simulink model "s_heli3d_Kalman_Filter"  (Simulink 7.7)
settings: Solver=ode1  StartTime=0.0  StopTime=70  FixedStep=0.007  RelTol=1e-3
values from neighbouring files (symbols this model uses):
  A = double(subs(J_a,{'x1','x2','x3','x4','x5','x6','u1','u2'},{x0(1),x0(2),x0(3),x0(4),x0(5),x0(6),u0(1),u0(2)}))    [linnlsys.m]    (also in o_lqi.m = A_lin)
  A_kal = Kest.a    [setup_lab_heli_3d_various_controler_with_Kalman_Filter.m]
  B = double(subs(J_b,{'x1','x2','x3','x4','x5','x6','u1','u2'},{x0(1),x0(2),x0(3),x0(4),x0(5),x0(6),u0(1),u0(2)}))    [linnlsys.m]    (also in o_lqi.m = B_lin)
  B_kal = Kest.b    [setup_lab_heli_3d_various_controler_with_Kalman_Filter.m]
  C_kal = eye(6)    [setup_lab_heli_3d_various_controler_with_Kalman_Filter.m]
  CMD_RATE_LIMIT = 45.0 * pi / 180    (= 0.785398163397)    [setup_lab_heli_3d.m]    (also in setup_lab_heli_3d_simple.m; setup_lab_heli_3d_various_controler.m; setup_lab_heli_3d_various_controler_with_Kalman_Filter.m)
  D_kal = zeros(6,5)    [setup_lab_heli_3d_various_controler_with_Kalman_Filter.m]
  K = lqr(A,B,Q_x,Q_u)    [lab_init.m]    (also in setup_lab_heli_3d.m = zeros(2,6); setup_lab_heli_3d_various_controler.m = lqr( Ai, Bi, Q, R ); setup_lab_heli_3d_various_controler_with_Kalman_Filter.m = lqr( Ai, Bi, Q, R ))
  K_AMP = 3    [setup_lab_heli_3d.m]    (also in setup_lab_heli_3d_simple.m; setup_lab_heli_3d_various_controler.m; setup_lab_heli_3d_various_controler_with_Kalman_Filter.m)
  SAT_INT_ERR_ELEV = 7.5    [setup_lab_heli_3d.m]    (also in setup_lab_heli_3d_simple.m; setup_lab_heli_3d_various_controler.m; setup_lab_heli_3d_various_controler_with_Kalman_Filter.m)
  SAT_INT_ERR_TRAVEL = 7.5    [setup_lab_heli_3d.m]    (also in setup_lab_heli_3d_simple.m; setup_lab_heli_3d_various_controler.m; setup_lab_heli_3d_various_controler_with_Kalman_Filter.m)
  VMAX_AMP = 24    [setup_lab_heli_3d.m]    (also in setup_lab_heli_3d_simple.m; setup_lab_heli_3d_various_controler.m; setup_lab_heli_3d_various_controler_with_Kalman_Filter.m)
  VMAX_DAC = 10    [setup_lab_heli_3d.m]    (also in setup_lab_heli_3d_simple.m; setup_lab_heli_3d_various_controler.m; setup_lab_heli_3d_various_controler_with_Kalman_Filter.m)
libraries: simulink_extras x3
settings Model: Creator=MLevis  LastModifiedBy=signaler  ExtModeTrigDuration=5000  ExtModeArmWhenConnect=off  BufferReuse=off
settings SolverCC: PositivePriorityOrder=on
settings OptimizationCC: BooleanDataType=off  InlineInvariantSignals=on  OptimizeBlockIOStorage=off  BufferReuse=off  ExpressionFolding=off  LocalBlockOutputs=off  InitFltsAndDblsToZero=on
settings DebuggingCC: SaveWithParameterizedLinksMsg=none  SignalResolutionControl=TryResolveAllWithWarning  MultiTaskDSMMsg=warning  MultiTaskCondExecSysMsg=none  StrictBusMsg=Warning
settings RTWCC: SystemTargetFile=quarc_windows.tlc  TemplateMakefile=quarc_default_tmf  Description=QUARC Win32 Target  ProcessScript=quarc_windows_make_rtw_hook  IncludeERTFirstTime=on
settings STFCustomTargetCC: TargetFcnLib=ansi_tfl_tmw.mat  TargetPreCompLibLocation=C:\PROGRA~3\QUARC\lib\2011a\windows\release  FunctionExecutionProfile=off  GeneratePreprocessorConditionals=Disable all  SystemTargetFile=quarc_windows.tlc
settings GRTTargetCC: TargetFcnLib=ansi_tfl_tmw.mat  TargetPreCompLibLocation=C:\PROGRA~3\QUARC\lib\2011a\windows\release  ParMdlRefBuildCompliant=off  CompOptLevelCompliant=off  MatFileLogging=off  ExtMode=on  ExtModeMexFile=quarc_comm

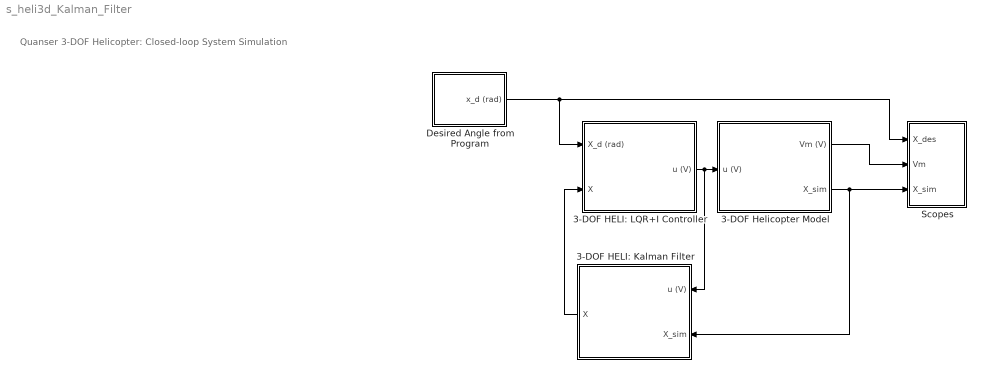
== system s_heli3d_Kalman_Filter ==
  note: Quanser 3-DOF Helicopter:
      | Closed-loop System Simulation
  3-DOF HELI: Kalman Filter : Subsystem  AncestorBlock=heli_2d_lib/2DOF HELI: FF+LQR+I Controller
  3-DOF HELI: LQR+I Controller : Subsystem  AncestorBlock=heli_2d_lib/2DOF HELI: FF+LQR+I Controller
  3-DOF Helicopter Model : Subsystem
  Desired Angle from Program : Subsystem
  Scopes : Subsystem
  wires:
  Desired Angle from Program/1(x_d (rad)) -> Scopes/1(X_des), 3-DOF HELI: LQR+I Controller/1(X_d (rad))
  3-DOF HELI: LQR+I Controller/1(u (V)) -> 3-DOF Helicopter Model/1(u (V)), 3-DOF HELI: Kalman Filter/1(u (V))
  3-DOF Helicopter Model/2(X_sim) -> Scopes/3(X_sim), 3-DOF HELI: Kalman Filter/2(X_sim)
  3-DOF Helicopter Model/1(Vm (V)) -> Scopes/2(Vm)
  3-DOF HELI: Kalman Filter/1(X) -> 3-DOF HELI: LQR+I Controller/2(X)

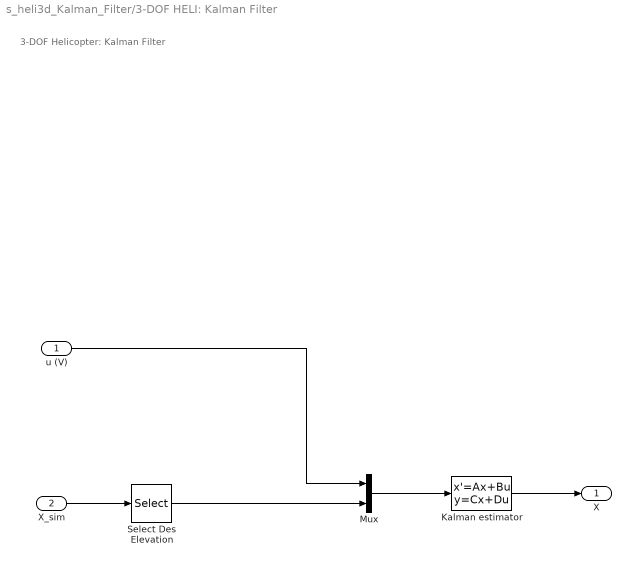
== system s_heli3d_Kalman_Filter/3-DOF HELI: Kalman Filter ==
  note: 3-DOF Helicopter: Kalman Filter
  u (V) : Inport
  X_sim : Inport  Port=2
  Kalman estimator : StateSpace  A=A_kal  B=B_kal  C=C_kal  D=D_kal
  Mux : Mux  Inputs=2
  Select Des Elevation : Selector  InputPortWidth=6  IndexOptions=Index vector (dialog)  Indices=[1:3]  OutputSizes=1
  X : Outport
  wires:
  Mux/1 -> Kalman estimator/1
  Select Des Elevation/1 -> Mux/2
  u (V)/1 -> Mux/1
  Kalman estimator/1 -> X/1
  X_sim/1 -> Select Des Elevation/1

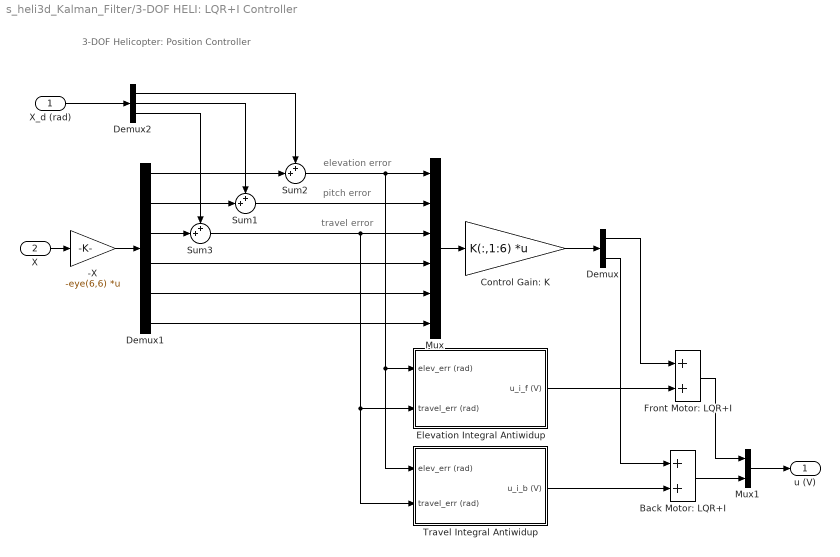
== system s_heli3d_Kalman_Filter/3-DOF HELI: LQR+I Controller ==
  note: elevation error
  note: pitch error
  note: 3-DOF Helicopter: Position Controller
  note: travel error
  X_d (rad) : Inport
  X : Inport  Port=2
  -X : Gain  Gain=-eye(6,6)  Multiplication=Matrix(K*u)
  Back Motor: LQR+I : Sum
  Control Gain: K : Gain  Gain=K(:,1:6)  Multiplication=Matrix(K*u)
  Demux : Demux  Outputs=2
  Demux1 : Demux  Outputs=6
  Demux2 : Demux  Outputs=3
  Elevation Integral Antiwidup : Subsystem
  Front Motor: LQR+I : Sum
  Mux : Mux  Inputs=6
  Mux1 : Mux  Inputs=2
  Sum1 : Sum  Inputs=++|
  Sum2 : Sum  Inputs=++|
  Sum3 : Sum  Inputs=++|
  Travel Integral Antiwidup : Subsystem
  u (V) : Outport
  wires:
  Back Motor: LQR+I/1 -> Mux1/2
  Demux/1 -> Front Motor: LQR+I/1
  Demux/2 -> Back Motor: LQR+I/1
  Travel Integral Antiwidup/1(u_i_b (V)) -> Back Motor: LQR+I/2
  Elevation Integral Antiwidup/1(u_i_f (V)) -> Front Motor: LQR+I/2
  Demux1/2 -> Sum1/2
  Demux2/2 -> Sum1/1
  Demux2/1 -> Sum2/1
  X_d (rad)/1 -> Demux2/1
  Sum2/1 -> Mux/1, Elevation Integral Antiwidup/1(elev_err (rad)), Travel Integral Antiwidup/1(elev_err (rad))
  Demux1/1 -> Sum2/2
  X/1 -> -X/1
  Sum1/1 -> Mux/2
  -X/1 -> Demux1/1
  Mux/1 -> Control Gain: K/1
  Demux1/4 -> Mux/4
  Demux2/3 -> Sum3/1
  Demux1/3 -> Sum3/2
  Sum3/1 -> Mux/3, Elevation Integral Antiwidup/2(travel_err (rad)), Travel Integral Antiwidup/2(travel_err (rad))
  Demux1/5 -> Mux/5
  Demux1/6 -> Mux/6
  Control Gain: K/1 -> Demux/1
  Mux1/1 -> u (V)/1
  Front Motor: LQR+I/1 -> Mux1/1

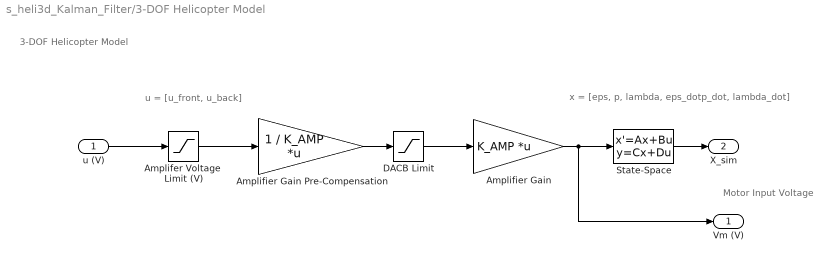
== system s_heli3d_Kalman_Filter/3-DOF Helicopter Model ==
  note: x = [eps, p, lambda, eps_dotp_dot, lambda_dot]
  note: u = [u_front, u_back]
  note: Motor Input Voltage
  note: 3-DOF Helicopter Model
  u (V) : Inport
  Amplifer Voltage  Limit (V) : Saturate  UpperLimit=VMAX_AMP  LowerLimit=-VMAX_AMP
  Amplifier Gain : Gain  Gain=K_AMP  Multiplication=Matrix(K*u)  SaturateOnIntegerOverflow=on  OutDataTypeStr=Inherit: Same as input  ParamDataTypeStr=Inherit: Same as input
  Amplifier Gain Pre-Compensation : Gain  Gain=1 / K_AMP  Multiplication=Matrix(K*u)  SaturateOnIntegerOverflow=on  OutDataTypeStr=Inherit: Same as input  ParamDataTypeStr=Inherit: Same as input
  DACB Limit : Saturate  UpperLimit=VMAX_DAC  LowerLimit=-VMAX_DAC
  State-Space : StateSpace  A=A  B=B  C=eye(6,6)  D=zeros(6,2)
  Vm (V) : Outport
  X_sim : Outport  Port=2
  wires:
  u (V)/1 -> Amplifer Voltage  Limit (V)/1
  Amplifier Gain/1 -> Vm (V)/1, State-Space/1
  State-Space/1 -> X_sim/1
  Amplifer Voltage  Limit (V)/1 -> Amplifier Gain Pre-Compensation/1
  Amplifier Gain Pre-Compensation/1 -> DACB Limit/1
  DACB Limit/1 -> Amplifier Gain/1

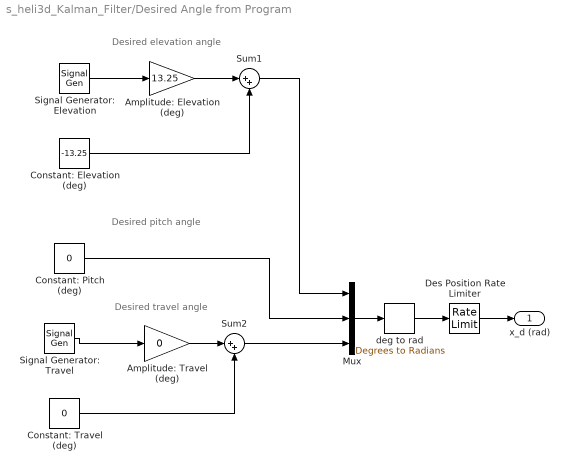
== system s_heli3d_Kalman_Filter/Desired Angle from Program ==
  note: Desired elevation angle
  note: Desired travel angle
  note: Desired pitch angle
  Amplitude: Elevation (deg) : Gain  Gain=13.25
  Amplitude: Travel (deg) : Gain  Gain=0
  Constant: Elevation (deg) : Constant  Value=-13.25
  Constant: Pitch (deg) : Constant  Value=0
  Constant: Travel (deg) : Constant  Value=0
  Des Position Rate Limiter : RateLimiter  RisingSlewLimit=CMD_RATE_LIMIT  FallingSlewLimit=-CMD_RATE_LIMIT  SampleTimeMode=inherited
  Mux : Mux  Inputs=3
  Signal Generator: Elevation : SignalGenerator  WaveForm=square  Frequency=0.01
  Signal Generator: Travel : SignalGenerator  Frequency=0.02
  Sum1 : Sum  Inputs=|++
  Sum2 : Sum  Inputs=|++
  deg to rad : simulink_extras/Transformations/Degrees to Radians  SystemSampleTime=-1
  x_d (rad) : Outport
  wires:
  Mux/1 -> deg to rad/1
  Constant: Elevation (deg)/1 -> Sum1/2
  Amplitude: Elevation (deg)/1 -> Sum1/1
  Signal Generator: Elevation/1 -> Amplitude: Elevation (deg)/1
  Constant: Travel (deg)/1 -> Sum2/2
  Amplitude: Travel (deg)/1 -> Sum2/1
  Signal Generator: Travel/1 -> Amplitude: Travel (deg)/1
  Sum2/1 -> Mux/3
  deg to rad/1 -> Des Position Rate Limiter/1
  Constant: Pitch (deg)/1 -> Mux/2
  Sum1/1 -> Mux/1
  Des Position Rate Limiter/1 -> x_d (rad)/1

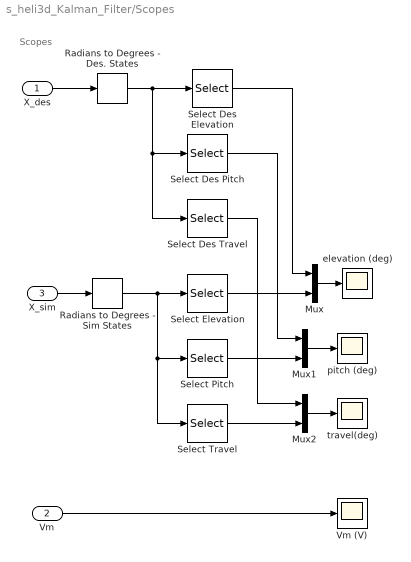
== system s_heli3d_Kalman_Filter/Scopes ==
  note: Scopes
  X_des : Inport
  Vm : Inport  Port=2
  X_sim : Inport  Port=3
  Mux : Mux  Inputs=2
  Mux1 : Mux  Inputs=2
  Mux2 : Mux  Inputs=2
  Radians to Degrees - Des. States : simulink_extras/Transformations/Radians to Degrees  SystemSampleTime=-1
  Radians to Degrees - Sim States : simulink_extras/Transformations/Radians to Degrees  SystemSampleTime=-1
  Select Des Elevation : Selector  InputPortWidth=3  IndexOptions=Index vector (dialog)  Indices=1  OutputSizes=1
  Select Des Pitch : Selector  InputPortWidth=3  IndexOptions=Index vector (dialog)  Indices=2  OutputSizes=1
  Select Des Travel : Selector  InputPortWidth=3  IndexOptions=Index vector (dialog)  Indices=3  OutputSizes=1
  Select Elevation : Selector  InputPortWidth=6  IndexOptions=Index vector (dialog)  Indices=1  OutputSizes=1
  Select Pitch : Selector  InputPortWidth=6  IndexOptions=Index vector (dialog)  Indices=2  OutputSizes=1
  Select Travel : Selector  InputPortWidth=6  IndexOptions=Index vector (dialog)  Indices=3  OutputSizes=1
  Vm (V) : Scope
      settings: TickLabels=on  TimeRange=60  YMin=-25  YMax=25  SaveName=ScopeData4  DataFormat=Array
  elevation (deg) : Scope
      settings: TickLabels=on  TimeRange=70  YMin=-15  YMax=15  DataFormat=Array
  pitch (deg) : Scope
      settings: TickLabels=on  TimeRange=60  YMin=-30  YMax=30  DataFormat=Array
  travel(deg) : Scope
      settings: TickLabels=on  TimeRange=60  YMin=-100  YMax=100  SaveName=ScopeData2  DataFormat=Array
  wires:
  X_des/1 -> Radians to Degrees - Des. States/1
  X_sim/1 -> Radians to Degrees - Sim States/1
  Mux/1 -> elevation (deg)/1
  Mux1/1 -> pitch (deg)/1
  Vm/1 -> Vm (V)/1
  Radians to Degrees - Sim States/1 -> Select Elevation/1, Select Pitch/1, Select Travel/1
  Mux2/1 -> travel(deg)/1
  Select Elevation/1 -> Mux/2
  Select Pitch/1 -> Mux1/2
  Select Travel/1 -> Mux2/2
  Radians to Degrees - Des. States/1 -> Select Des Elevation/1, Select Des Pitch/1, Select Des Travel/1
  Select Des Elevation/1 -> Mux/1
  Select Des Pitch/1 -> Mux1/1
  Select Des Travel/1 -> Mux2/1

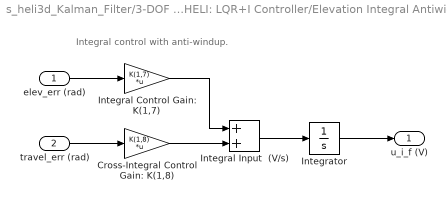
== system s_heli3d_Kalman_Filter/3-DOF HELI: LQR+I Controller/Elevation Integral Antiwidup ==
  note: Integral control with anti-windup.
  elev_err (rad) : Inport
  travel_err (rad) : Inport  Port=2
  Cross-Integral Control Gain: K(1,8) : Gain  Gain=K(1,8)  Multiplication=Matrix(K*u)
  Integral Control Gain: K(1,7) : Gain  Gain=K(1,7)  Multiplication=Matrix(K*u)
  Integral Input  (V/s) : Sum
  Integrator : Integrator  LimitOutput=on  UpperSaturationLimit=SAT_INT_ERR_ELEV  LowerSaturationLimit=-SAT_INT_ERR_ELEV
  u_i_f (V) : Outport
  wires:
  Cross-Integral Control Gain: K(1,8)/1 -> Integral Input  (V/s)/2
  Integral Control Gain: K(1,7)/1 -> Integral Input  (V/s)/1
  travel_err (rad)/1 -> Cross-Integral Control Gain: K(1,8)/1
  elev_err (rad)/1 -> Integral Control Gain: K(1,7)/1
  Integral Input  (V/s)/1 -> Integrator/1
  Integrator/1 -> u_i_f (V)/1

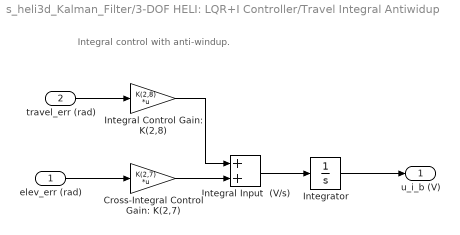
== system s_heli3d_Kalman_Filter/3-DOF HELI: LQR+I Controller/Travel Integral Antiwidup ==
  note: Integral control with anti-windup.
  elev_err (rad) : Inport
  travel_err (rad) : Inport  Port=2
  Cross-Integral Control Gain: K(2,7) : Gain  Gain=K(2,7)  Multiplication=Matrix(K*u)
  Integral Control Gain: K(2,8) : Gain  Gain=K(2,8)  Multiplication=Matrix(K*u)
  Integral Input  (V/s) : Sum
  Integrator : Integrator  LimitOutput=on  UpperSaturationLimit=SAT_INT_ERR_TRAVEL  LowerSaturationLimit=-SAT_INT_ERR_TRAVEL
  u_i_b (V) : Outport
  wires:
  Cross-Integral Control Gain: K(2,7)/1 -> Integral Input  (V/s)/2
  Integral Control Gain: K(2,8)/1 -> Integral Input  (V/s)/1
  travel_err (rad)/1 -> Integral Control Gain: K(2,8)/1
  elev_err (rad)/1 -> Cross-Integral Control Gain: K(2,7)/1
  Integral Input  (V/s)/1 -> Integrator/1
  Integrator/1 -> u_i_b (V)/1
